simulink model "ugvGNC_complete"  (R2019a)
settings: Solver=ode45  StartTime=0.0  StopTime=200  RelTol=1e-3
InitFcn:
  | UGVparameters
StopFcn:
  | myPlot(xActEst,yActEst,X_array,Y_array,rp1,rp2)
values from neighbouring files (symbols this model uses):
  b = 0.5842    [GNCparameters.m]
  bDR = b    (= 0.5842)    [GNCparameters.m]
  eTick = 900    [GNCparameters.m]
  KP1 = 10    [GNCparameters.m]
  KP2 = 10    [GNCparameters.m]
  rL = 0.052959    [GNCparameters.m]
  rp1 = 0.3    [GNCparameters.m]
  rp2 = 0.5    [GNCparameters.m]
  rR = 0.052959    [GNCparameters.m]
  Tau1 = 0.01    [GNCparameters.m]
  Tau2 = 0.1    [GNCparameters.m]
  TauEncoderDR = 0.1    [GNCparameters.m]
  Tsample = 1/10    (= 0.1)    [GNCparameters.m]
  TsampleEncoder = 0.1    [GNCparameters.m]
  TsampleEncoderDR = TsampleEncoder    (= 0.1)    [GNCparameters.m]
  Vcom = 3*Vmax/4    (= 0.33)    [GNCparameters.m]
  wmax = Vmax/rR    (= 8.30831397874)    [GNCparameters.m]
  X_array = [3 6 6 3 0 0]    [GNCparameters.m]
  Y_array = [5 0 13 8 13 0]    [GNCparameters.m]
undefined symbols (not defined in the file or in its folder): DiscIntNeverNeededParam
libraries: simulink x12
settings Model: Creator=vigal  LastModifiedBy=lalit
settings DataIOCC: ReturnWorkspaceOutputs=off
settings DebuggingCC: ArithmeticOperatorsInVariantConditions=warning
settings SFSimCC: SimUseLocalCustomCode=off
settings RTWCC: RTWUseLocalCustomCode=off

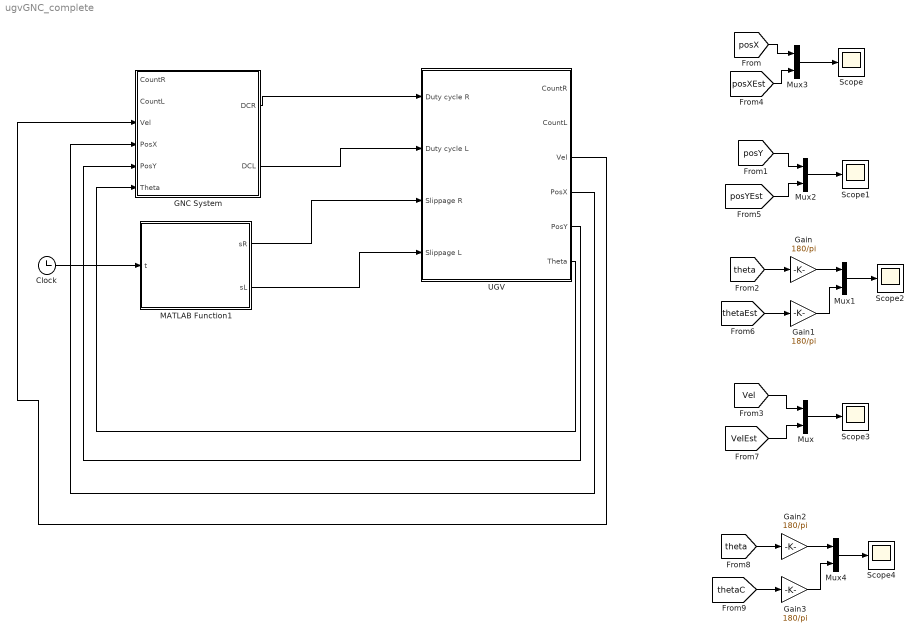
== system ugvGNC_complete ==
  Clock : Clock
  GNC System : Subsystem
  Gain{,1..3} (4 alike) : Gain  Gain=180/pi
  MATLAB Function1 : MATLAB Function  TreatAsAtomicUnit=on
  Mux{,1..4} (5 alike) : Mux  Inputs=2
  Scope{,1..4} (5 alike) : Scope
  UGV : Subsystem
  wires:
  Clock/1 -> MATLAB Function1/1(t)
  MATLAB Function1/1(sR) -> UGV/3(Slippage R)
  MATLAB Function1/2(sL) -> UGV/4(Slippage L)
  [theta] -> Gain/1
  [posX] -> Mux3/1
  [posXEst] -> Mux3/2
  Mux3/1 -> Scope/1
  Mux2/1 -> Scope1/1
  [posY] -> Mux2/1
  [posYEst] -> Mux2/2
  Gain/1 -> Mux1/1
  Mux1/1 -> Scope2/1
  [thetaEst] -> Gain1/1
  [Vel] -> Mux/1
  [VelEst] -> Mux/2
  Mux/1 -> Scope3/1
  Gain1/1 -> Mux1/2
  GNC System/1(DCR) -> UGV/1(Duty cycle R)
  GNC System/2(DCL) -> UGV/2(Duty cycle L)
  Gain3/1 -> Mux4/2
  [thetaC] -> Gain3/1
  Mux4/1 -> Scope4/1
  [theta] -> Gain2/1
  Gain2/1 -> Mux4/1
  UGV/3(Vel) -> GNC System/3(Vel)
  UGV/4(PosX) -> GNC System/4(PosX)
  UGV/5(PosY) -> GNC System/5(PosY)
  UGV/6(Theta) -> GNC System/6(Theta)

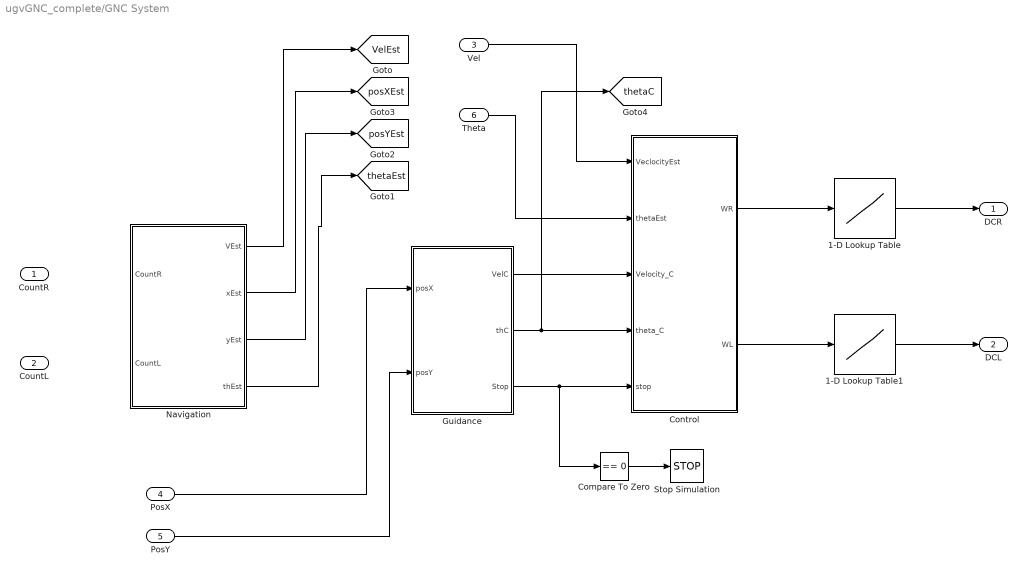
== system ugvGNC_complete/GNC System ==
  CountR : Inport
  CountL : Inport  Port=2
  Vel : Inport  Port=3
  PosX : Inport  Port=4
  PosY : Inport  Port=5
  Theta : Inport  Port=6
  1-D Lookup Table : Lookup_n-D  NumberOfTableDimensions=1  BreakpointsForDimension1=[-wmax -wmax/100 0 wmax/100 wmax]  Table=[-100 -30 0 30 100]  InternalRulePriority=Speed  RndMeth=Simplest  InputSameDT=on
  1-D Lookup Table1 : Lookup_n-D  NumberOfTableDimensions=1  BreakpointsForDimension1=[-wmax -wmax/100 0 wmax/100 wmax]  Table=[-100 -30 0 30 100]  InternalRulePriority=Speed  RndMeth=Simplest  InputSameDT=on
  Compare To Zero : simulink/Logic and Bit Operations/Compare To Zero  relop===  OutDataTypeStr=boolean
  Control : Subsystem
  Guidance : Subsystem
  Navigation : Subsystem
  Stop Simulation : Stop
  DCR : Outport
  DCL : Outport  Port=2
  tag scope: VelEst=global, posXEst=global, posYEst=global, thetaC=global, thetaEst=global
  wires:
  Navigation/1(VEst) -> [VelEst]
  Navigation/2(xEst) -> [posXEst]
  Navigation/3(yEst) -> [posYEst]
  Navigation/4(thEst) -> [thetaEst]
  Guidance/1(VelC) -> Control/3(Velocity_C)
  Guidance/2(thC) -> [thetaC], Control/4(theta_C)
  Guidance/3(Stop) -> Compare To Zero/1, Control/5(stop)
  Control/1(WR) -> 1-D Lookup Table/1
  Control/2(WL) -> 1-D Lookup Table1/1
  Compare To Zero/1 -> Stop Simulation/1
  PosX/1 -> Guidance/1(posX)
  PosY/1 -> Guidance/2(posY)
  Theta/1 -> Control/2(thetaEst)
  Vel/1 -> Control/1(VeclocityEst)
  1-D Lookup Table/1 -> DCR/1
  1-D Lookup Table1/1 -> DCL/1

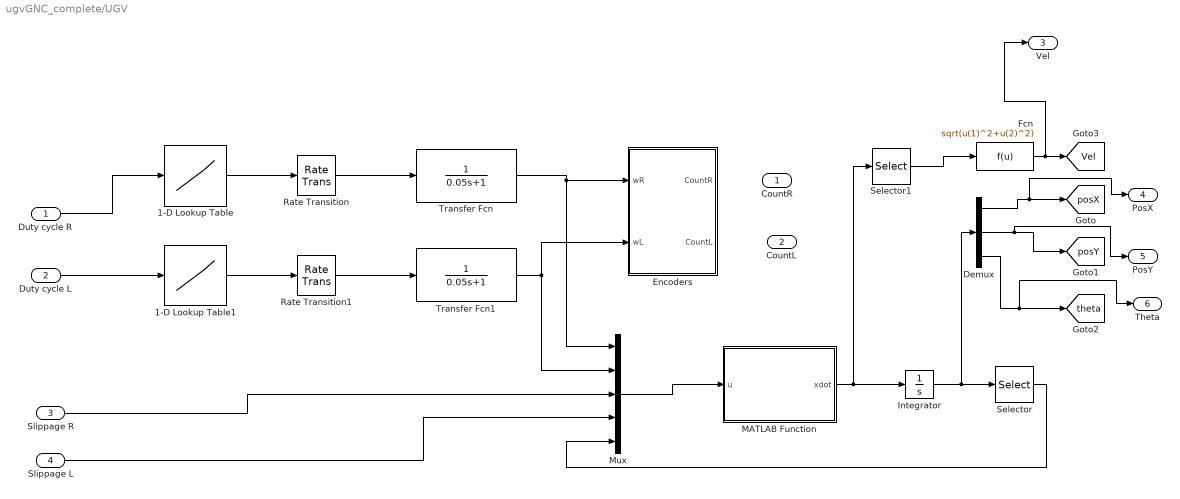
== system ugvGNC_complete/UGV ==
  Duty cycle R : Inport
  Duty cycle L : Inport  Port=2
  Slippage R : Inport  Port=3
  Slippage L : Inport  Port=4
  1-D Lookup Table : Lookup_n-D  NumberOfTableDimensions=1  BreakpointsForDimension1=[-100 -30 0 30 100]  Table=[-wmax 0 0 0 wmax]  InternalRulePriority=Speed  RndMeth=Simplest  InputSameDT=on
  1-D Lookup Table1 : Lookup_n-D  NumberOfTableDimensions=1  BreakpointsForDimension1=[-100 -30 0 30 100]  Table=[-wmax 0 0 0 wmax]  InternalRulePriority=Speed  RndMeth=Simplest  InputSameDT=on
  Demux : Demux  Outputs=3
  Encoders : Subsystem
  Fcn : Fcn  Expr=sqrt(u(1)^2+u(2)^2)
  Integrator : Integrator  InitialCondition=[0;0;0]
  MATLAB Function : MATLAB Function  TreatAsAtomicUnit=on
  Mux : Mux  Inputs=5
  Rate Transition : RateTransition
  Rate Transition1 : RateTransition
  Selector : Selector  InputPortWidth=3  IndexOptions=Index vector (dialog)  Indices=[3]  OutputSizes=1
  Selector1 : Selector  InputPortWidth=3  IndexOptions=Index vector (dialog)  Indices=[1 2]  OutputSizes=1
  Transfer Fcn : TransferFcn  Denominator=[0.05 1]
  Transfer Fcn1 : TransferFcn  Denominator=[0.05 1]
  CountR : Outport
  CountL : Outport  Port=2
  Vel : Outport  Port=3
  PosX : Outport  Port=4
  PosY : Outport  Port=5
  Theta : Outport  Port=6
  tag scope: Vel=global, posX=global, posY=global, theta=global
  wires:
  Slippage R/1 -> Mux/3
  1-D Lookup Table/1 -> Rate Transition/1
  Duty cycle R/1 -> 1-D Lookup Table/1
  Duty cycle L/1 -> 1-D Lookup Table1/1
  1-D Lookup Table1/1 -> Rate Transition1/1
  Rate Transition1/1 -> Transfer Fcn1/1
  Rate Transition/1 -> Transfer Fcn/1
  Transfer Fcn/1 -> Encoders/1(wR), Mux/1
  Slippage L/1 -> Mux/4
  Transfer Fcn1/1 -> Encoders/2(wL), Mux/2
  Mux/1 -> MATLAB Function/1(u)
  Integrator/1 -> Demux/1, Selector/1
  Selector/1 -> Mux/5
  Demux/1 -> PosX/1, [posX]
  Demux/3 -> Theta/1, [theta]
  Demux/2 -> PosY/1, [posY]
  MATLAB Function/1(xdot) -> Selector1/1, Integrator/1
  Selector1/1 -> Fcn/1
  Fcn/1 -> Vel/1, [Vel]

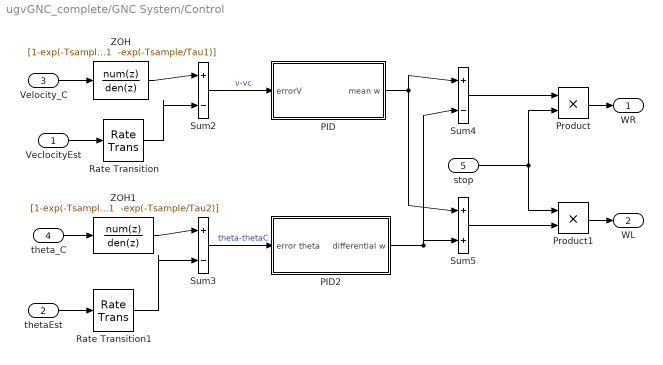
== system ugvGNC_complete/GNC System/Control ==
  VeclocityEst : Inport
  thetaEst : Inport  Port=2
  Velocity_C : Inport  Port=3
  theta_C : Inport  Port=4
  stop : Inport  Port=5
  PID : Subsystem
  PID2 : Subsystem
  Product : Product  RndMeth=Zero
  Product1 : Product  RndMeth=Zero
  Rate Transition : RateTransition  Deterministic=off
  Rate Transition1 : RateTransition  Deterministic=off
  Sum2 : Sum  Inputs=|+|-|  SampleTime=Tsample
  Sum3 : Sum  Inputs=|+|-|  SampleTime=Tsample
  Sum4 : Sum  Inputs=+|-
  Sum5 : Sum  Inputs=+|+
  ZOH : DiscreteTransferFcn  Numerator=[1-exp(-Tsample/Tau1)]  Denominator="[1  -exp(-Tsample/Tau1)]"  SampleTime=Tsample
  ZOH1 : DiscreteTransferFcn  Numerator=[1-exp(-Tsample/Tau2)]  Denominator="[1  -exp(-Tsample/Tau2)]"  SampleTime=Tsample
  WR : Outport
  WL : Outport  Port=2
  wires:
  Product1/1 -> WL/1
  Product/1 -> WR/1
  Sum5/1 -> Product1/2
  stop/1 -> Product/2, Product1/1
  Sum4/1 -> Product/1
  PID2/1(differential w) -> Sum5/2, Sum4/2
  PID/1(mean w) -> Sum5/1, Sum4/1
  theta_C/1 -> ZOH1/1
  thetaEst/1 -> Rate Transition1/1
  Velocity_C/1 -> ZOH/1
  VeclocityEst/1 -> Rate Transition/1
  Sum2/1 -> PID/1(errorV)  "v-vc"
  Sum3/1 -> PID2/1(error theta)  "theta-thetaC"
  ZOH/1 -> Sum2/1
  Rate Transition/1 -> Sum2/2
  ZOH1/1 -> Sum3/1
  Rate Transition1/1 -> Sum3/2

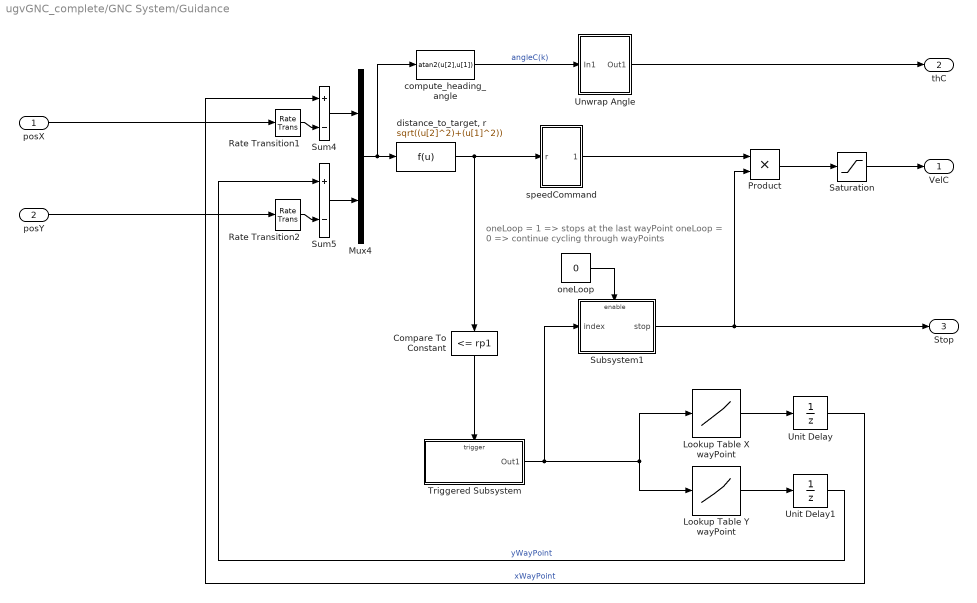
== system ugvGNC_complete/GNC System/Guidance ==
  note: oneLoop = 1 => stops at the last wayPoint
      | oneLoop = 0 => continue cycling through wayPoints
  posX : Inport
  posY : Inport  Port=2
  Compare To Constant : simulink/Logic and Bit Operations/Compare To Constant  relop=<=  const=rp1  OutDataTypeStr=uint8  ZeroCross=off
  Lookup Table X wayPoint : Lookup  InputValues=[1:length(X_array)]  Table=X_array  LookUpMeth=Interpolation-Use End Values  OutDataTypeStr=double
  Lookup Table Y wayPoint : Lookup  InputValues=[1:length(Y_array)]  Table=Y_array  LookUpMeth=Interpolation-Use End Values  OutDataTypeStr=double
  Mux4 : Mux  Inputs=2
  Product : Product  RndMeth=Zero
  Rate Transition1 : RateTransition
  Rate Transition2 : RateTransition
  Saturation : Saturate  UpperLimit=Vcom  LowerLimit=0  SampleTime=Tsample
  Subsystem1 : Subsystem
  Sum4 : Sum  Inputs=|+|-|
  Sum5 : Sum  Inputs=|+|-|
  Triggered Subsystem : Subsystem  TreatAsAtomicUnit=on
  Unit Delay : UnitDelay  SampleTime=Tsample  HasFrameUpgradeWarning=on
  Unit Delay1 : UnitDelay  SampleTime=Tsample  HasFrameUpgradeWarning=on
  Unwrap Angle : Subsystem
  compute_heading_angle : Fcn  Expr=atan2(u[2],u[1])  SampleTime=Tsample
  "distance_to_target, r" : Fcn  Expr=sqrt((u[2]^2)+(u[1]^2))  SampleTime=Tsample
  oneLoop : Constant  Value=0  OutDataTypeStr=uint32  SampleTime=Tsample
  speedCommand : Subsystem
  VelC : Outport
  thC : Outport  Port=2
  Stop : Outport  Port=3
  wires:
  Compare To Constant/1 -> Triggered Subsystem/Trigger
  oneLoop/1 -> Subsystem1/Enable
  Sum5/1 -> Mux4/2
  Unit Delay/1 -> Sum4/1  "xWayPoint"
  Triggered Subsystem/1(Out1) -> Subsystem1/1(index), Lookup Table X wayPoint/1, Lookup Table Y wayPoint/1
  Lookup Table Y wayPoint/1 -> Unit Delay1/1
  Sum4/1 -> Mux4/1
  Subsystem1/1(stop) -> Stop/1, Product/2
  Product/1 -> Saturation/1
  Rate Transition1/1 -> Sum4/2
  Unit Delay1/1 -> Sum5/1  "yWayPoint"
  posX/1 -> Rate Transition1/1
  posY/1 -> Rate Transition2/1
  Mux4/1 -> "distance_to_target, r"/1, compute_heading_angle/1
  Lookup Table X wayPoint/1 -> Unit Delay/1
  Rate Transition2/1 -> Sum5/2
  compute_heading_angle/1 -> Unwrap Angle/1(In1)  "angleC(k)"
  "distance_to_target, r"/1 -> Compare To Constant/1, speedCommand/1(r)
  speedCommand/1(Vdes) -> Product/1
  Saturation/1 -> VelC/1
  Unwrap Angle/1(Out1) -> thC/1

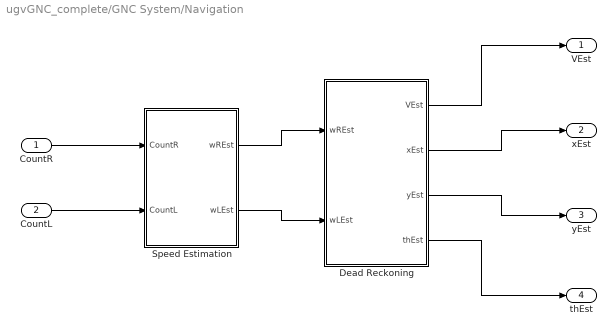
== system ugvGNC_complete/GNC System/Navigation ==
  CountR : Inport
  CountL : Inport  Port=2
  Dead Reckoning : Subsystem
  Speed Estimation : Subsystem
  VEst : Outport
  xEst : Outport  Port=2
  yEst : Outport  Port=3
  thEst : Outport  Port=4
  wires:
  Dead Reckoning/1(VEst) -> VEst/1
  Dead Reckoning/3(yEst) -> yEst/1
  Speed Estimation/2(wLEst) -> Dead Reckoning/2(wLEst)
  CountR/1 -> Speed Estimation/1(CountR)
  Dead Reckoning/2(xEst) -> xEst/1
  CountL/1 -> Speed Estimation/2(CountL)
  Speed Estimation/1(wREst) -> Dead Reckoning/1(wREst)
  Dead Reckoning/4(thEst) -> thEst/1

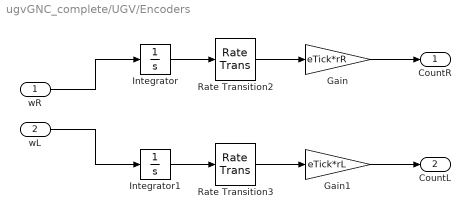
== system ugvGNC_complete/UGV/Encoders ==
  wR : Inport
  wL : Inport  Port=2
  Gain : Gain  Gain=eTick*rR  OutDataTypeStr=int16
  Gain1 : Gain  Gain=eTick*rL  OutDataTypeStr=int16
  Integrator : Integrator
  Integrator1 : Integrator
  Rate Transition2 : RateTransition  OutPortSampleTime=TsampleEncoder
  Rate Transition3 : RateTransition  OutPortSampleTime=TsampleEncoder
  CountR : Outport
  CountL : Outport  Port=2
  wires:
  Integrator1/1 -> Rate Transition3/1
  Integrator/1 -> Rate Transition2/1
  Gain1/1 -> CountL/1
  Rate Transition3/1 -> Gain1/1
  Rate Transition2/1 -> Gain/1
  Gain/1 -> CountR/1
  wR/1 -> Integrator/1
  wL/1 -> Integrator1/1

== system ugvGNC_complete/GNC System/Control/PID ==
  errorV : Inport
  Discrete Derivative : simulink/Discrete/Discrete Derivative  gainval=KD1  ICPrevScaledInput=0.0  OutMin=[]  OutMax=[]  OutDataType=sfix(16)  OutScaling=2^-10  DoSatur=off
  Discrete-Time Integrator : DiscreteIntegrator  gainval=KI1  SampleTime=Tsample  ICPrevOutput=DiscIntNeverNeededParam  ICPrevScaledInput=DiscIntNeverNeededParam
  Gain : Gain  Gain=KP1  SampleTime=Tsample
  Sum : Sum  Inputs=+|+|+
  Zero-Order Hold : ZeroOrderHold  SampleTime=Tsample
  mean w : Outport
  wires:
  Discrete Derivative/1 -> Sum/3
  Zero-Order Hold/1 -> Discrete Derivative/1
  Discrete-Time Integrator/1 -> Sum/2
  Gain/1 -> Sum/1
  errorV/1 -> Discrete-Time Integrator/1, Gain/1, Zero-Order Hold/1
  Sum/1 -> mean w/1

== system ugvGNC_complete/GNC System/Control/PID2 ==
  error theta : Inport
  Discrete Derivative1 : simulink/Discrete/Discrete Derivative  gainval=KD2  ICPrevScaledInput=0.0  OutMin=[]  OutMax=[]  OutDataType=sfix(16)  OutScaling=2^-10  DoSatur=off
  Discrete-Time Integrator1 : DiscreteIntegrator  gainval=KI2  SampleTime=Tsample  ICPrevOutput=DiscIntNeverNeededParam  ICPrevScaledInput=DiscIntNeverNeededParam
  Gain1 : Gain  Gain=KP2  SampleTime=Tsample
  Sum1 : Sum  Inputs=+|+|+
  Zero-Order Hold1 : ZeroOrderHold  SampleTime=Tsample
  differential w : Outport
  wires:
  Discrete Derivative1/1 -> Sum1/3
  Zero-Order Hold1/1 -> Discrete Derivative1/1
  error theta/1 -> Gain1/1, Discrete-Time Integrator1/1, Zero-Order Hold1/1
  Discrete-Time Integrator1/1 -> Sum1/2
  Gain1/1 -> Sum1/1
  Sum1/1 -> differential w/1

== system ugvGNC_complete/GNC System/Guidance/Subsystem1 ==
  note: NAND = TRUE
      | if at least one input is FALSE
  index : Inport
  Enable : EnablePort
  Compare To Constant1 : simulink/Logic and Bit Operations/Compare To Constant  relop===  const=1  OutDataTypeStr=uint8  ZeroCross=off
  Compare To Constant2 : simulink/Logic and Bit Operations/Compare To Constant  relop===  const=length(X_array)  OutDataTypeStr=uint8  ZeroCross=off
  Logical Operator1 : Logic  Operator=NAND  IconShape=distinctive  AllPortsSameDT=off  OutDataTypeStr=boolean
  Triggered Subsystem2 : Subsystem  TreatAsAtomicUnit=on
  stop : Outport  OutputWhenDisabled=reset  InitialOutput=[1]
  wires:
  Logical Operator1/1 -> stop/1
  index/1 -> Compare To Constant1/1, Compare To Constant2/1
  Compare To Constant1/1 -> Logical Operator1/1
  Triggered Subsystem2/1(Out1) -> Logical Operator1/2
  Compare To Constant2/1 -> Triggered Subsystem2/Trigger

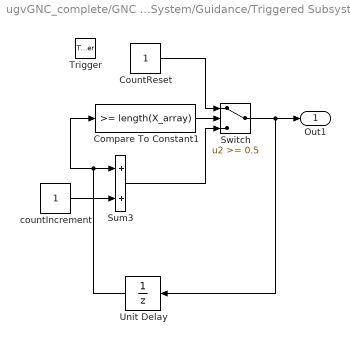
== system ugvGNC_complete/GNC System/Guidance/Triggered Subsystem ==
  Trigger : TriggerPort  VariantControl=(inherit)
  Compare To Constant1 : simulink/Logic and Bit Operations/Compare To Constant  relop=>=  const=length(X_array)  OutDataTypeStr=uint8  ZeroCross=off
  CountReset : Constant  OutDataTypeStr=uint32  SampleTime=-1
  Sum3 : Sum  OutDataTypeStr=uint32
  Switch : Switch  Threshold=0.5
  Unit Delay : UnitDelay  InitialCondition=1  SampleTime=-1  HasFrameUpgradeWarning=on
  countIncrement : Constant  OutDataTypeStr=uint32  SampleTime=-1
  Out1 : Outport  OutDataTypeStr=uint32  InitialOutput=1
  wires:
  countIncrement/1 -> Sum3/2
  Unit Delay/1 -> Compare To Constant1/1, Sum3/1
  Compare To Constant1/1 -> Switch/2
  Switch/1 -> Out1/1, Unit Delay/1
  CountReset/1 -> Switch/1
  Sum3/1 -> Switch/3

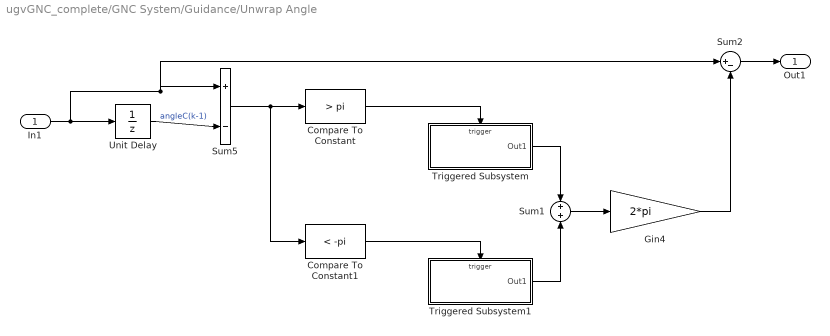
== system ugvGNC_complete/GNC System/Guidance/Unwrap Angle ==
  In1 : Inport
  Compare To Constant : simulink/Logic and Bit Operations/Compare To Constant  relop=>  const=pi  OutDataTypeStr=uint8  ZeroCross=off
  Compare To Constant1 : simulink/Logic and Bit Operations/Compare To Constant  relop=<  const=-pi  OutDataTypeStr=uint8  ZeroCross=off
  Gin4 : Gain  Gain=2*pi  OutDataTypeStr=double  SampleTime=Tsample
  Sum1 : Sum  Inputs=+|+
  Sum2 : Sum  Inputs=|+-
  Sum5 : Sum  Inputs=|+|-|
  Triggered Subsystem : Subsystem  TreatAsAtomicUnit=on
  Triggered Subsystem1 : Subsystem  TreatAsAtomicUnit=on
  Unit Delay : UnitDelay  SampleTime=Tsample  HasFrameUpgradeWarning=on
  Out1 : Outport
  wires:
  In1/1 -> Unit Delay/1, Sum5/1, Sum2/1
  Unit Delay/1 -> Sum5/2  "angleC(k-1)"
  Sum5/1 -> Compare To Constant/1, Compare To Constant1/1
  Compare To Constant1/1 -> Triggered Subsystem1/Trigger
  Compare To Constant/1 -> Triggered Subsystem/Trigger
  Triggered Subsystem/1(Out1) -> Sum1/1
  Triggered Subsystem1/1(Out1) -> Sum1/2
  Sum1/1 -> Gin4/1
  Sum2/1 -> Out1/1
  Gin4/1 -> Sum2/2

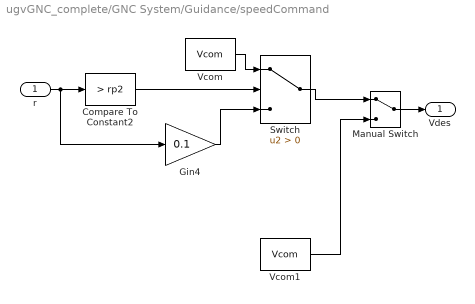
== system ugvGNC_complete/GNC System/Guidance/speedCommand ==
  r : Inport
  Compare To Constant2 : simulink/Logic and Bit Operations/Compare To Constant  relop=>  const=rp2  OutDataTypeStr=uint8  ZeroCross=off
  Gin4 : Gain  Gain=0.1  SampleTime=Tsample
  Manual Switch : ManualSwitch
  Switch : Switch  Criteria=u2 > Threshold
  Vcom : Constant  Value=Vcom  SampleTime=Tsample
  Vcom1 : Constant  Value=Vcom  SampleTime=Tsample
  Vdes : Outport
  wires:
  Compare To Constant2/1 -> Switch/2
  Vcom/1 -> Switch/1
  Vcom1/1 -> Manual Switch/2
  Switch/1 -> Manual Switch/1
  Gin4/1 -> Switch/3
  r/1 -> Compare To Constant2/1, Gin4/1
  Manual Switch/1 -> Vdes/1

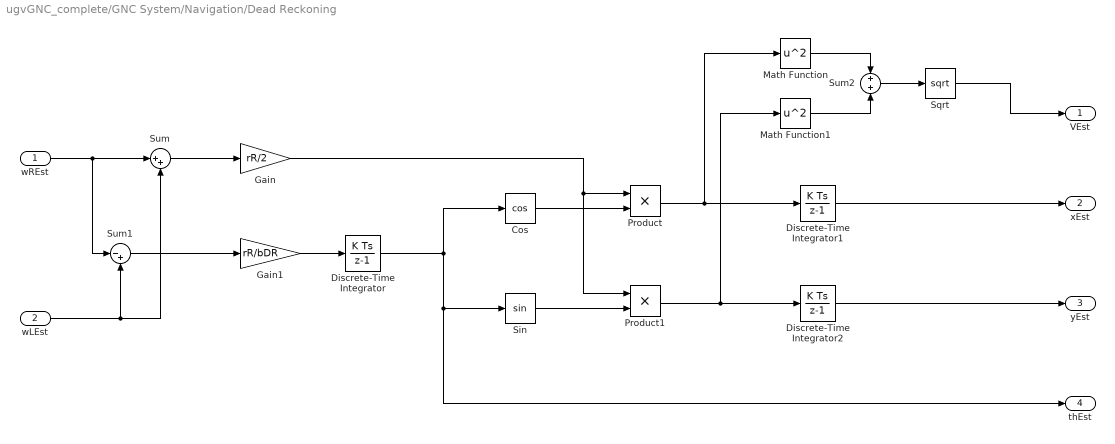
== system ugvGNC_complete/GNC System/Navigation/Dead Reckoning ==
  wREst : Inport
  wLEst : Inport  Port=2
  Cos : Trigonometry  Operator=cos
  Discrete-Time Integrator : DiscreteIntegrator  SampleTime=-1  OutDataTypeStr=double  ICPrevOutput=DiscIntNeverNeededParam  ICPrevScaledInput=DiscIntNeverNeededParam
  Discrete-Time Integrator1 : DiscreteIntegrator  SampleTime=-1  OutDataTypeStr=double  ICPrevOutput=DiscIntNeverNeededParam  ICPrevScaledInput=DiscIntNeverNeededParam
  Discrete-Time Integrator2 : DiscreteIntegrator  SampleTime=-1  OutDataTypeStr=double  ICPrevOutput=DiscIntNeverNeededParam  ICPrevScaledInput=DiscIntNeverNeededParam
  Gain : Gain  Gain=rR/2
  Gain1 : Gain  Gain=rR/bDR
  Math Function : Math  Operator=square  SaturateOnIntegerOverflow=on
  Math Function1 : Math  Operator=square  SaturateOnIntegerOverflow=on
  Product : Product
  Product1 : Product
  Sin : Trigonometry
  Sqrt : Sqrt  SaturateOnIntegerOverflow=on
  Sum : Sum  Inputs=|++
  Sum1 : Sum  Inputs=|-+
  Sum2 : Sum  Inputs=+|+
  VEst : Outport
  xEst : Outport  Port=2
  yEst : Outport  Port=3
  thEst : Outport  Port=4
  wires:
  wLEst/1 -> Sum1/2, Sum/2
  wREst/1 -> Sum1/1, Sum/1
  Sum/1 -> Gain/1
  Sum1/1 -> Gain1/1
  Gain1/1 -> Discrete-Time Integrator/1
  Discrete-Time Integrator/1 -> thEst/1, Sin/1, Cos/1
  Cos/1 -> Product/2
  Sin/1 -> Product1/2
  Gain/1 -> Product1/1, Product/1
  Product/1 -> Math Function/1, Discrete-Time Integrator1/1
  Product1/1 -> Math Function1/1, Discrete-Time Integrator2/1
  Math Function/1 -> Sum2/1
  Math Function1/1 -> Sum2/2
  Sum2/1 -> Sqrt/1
  Sqrt/1 -> VEst/1
  Discrete-Time Integrator1/1 -> xEst/1
  Discrete-Time Integrator2/1 -> yEst/1

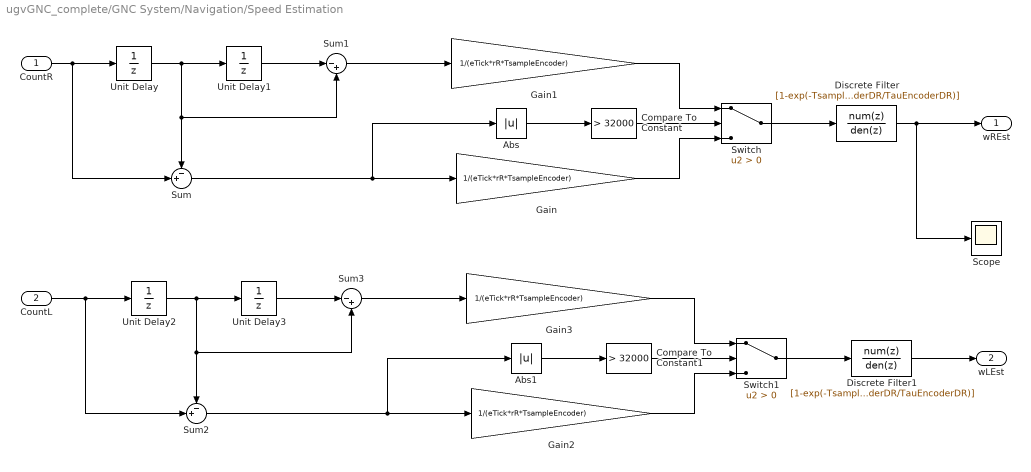
== system ugvGNC_complete/GNC System/Navigation/Speed Estimation ==
  CountR : Inport
  CountL : Inport  Port=2
  Abs : Abs
  Abs1 : Abs
  Compare To Constant : simulink/Logic and Bit Operations/Compare To Constant  relop=>  const=32000  OutDataTypeStr=boolean
  Compare To Constant1 : simulink/Logic and Bit Operations/Compare To Constant  relop=>  const=32000  OutDataTypeStr=boolean
  Discrete Filter : DiscreteFilter  Numerator=[1-exp(-TsampleEncoderDR/TauEncoderDR)]  Denominator=[1 -exp(-TsampleEncoderDR/TauEncoderDR)]
  Discrete Filter1 : DiscreteFilter  Numerator=[1-exp(-TsampleEncoderDR/TauEncoderDR)]  Denominator=[1 -exp(-TsampleEncoderDR/TauEncoderDR)]
  Gain{,1..3} (4 alike) : Gain  Gain=1/(eTick*rR*TsampleEncoder)
  Scope : Scope
  Sum : Sum  Inputs=-+|
  Sum1 : Sum  Inputs=|-+
  Sum2 : Sum  Inputs=-+|
  Sum3 : Sum  Inputs=|-+
  Switch : Switch  Criteria=u2 > Threshold
  Switch1 : Switch  Criteria=u2 > Threshold
  Unit Delay{,1..3} (4 alike) : UnitDelay  SampleTime=-1  HasFrameUpgradeWarning=on
  wREst : Outport
  wLEst : Outport  Port=2
  wires:
  Unit Delay/1 -> Sum1/2, Sum/1, Unit Delay1/1
  CountR/1 -> Sum/2, Unit Delay/1
  Unit Delay1/1 -> Sum1/1
  Sum/1 -> Abs/1, Gain/1
  Sum1/1 -> Gain1/1
  Abs/1 -> Compare To Constant/1
  Compare To Constant/1 -> Switch/2
  Gain/1 -> Switch/3
  Gain1/1 -> Switch/1
  Switch/1 -> Discrete Filter/1
  Discrete Filter/1 -> Scope/1, wREst/1
  Unit Delay2/1 -> Sum3/2, Sum2/1, Unit Delay3/1
  Unit Delay3/1 -> Sum3/1
  Sum3/1 -> Gain3/1
  CountL/1 -> Sum2/2, Unit Delay2/1
  Sum2/1 -> Abs1/1, Gain2/1
  Compare To Constant1/1 -> Switch1/2
  Discrete Filter1/1 -> wLEst/1
  Gain3/1 -> Switch1/1
  Switch1/1 -> Discrete Filter1/1
  Gain2/1 -> Switch1/3
  Abs1/1 -> Compare To Constant1/1

== system ugvGNC_complete/GNC System/Guidance/Subsystem1/Triggered Subsystem2 ==
  Trigger : TriggerPort  VariantControl=(inherit)
  Constant : Constant  OutDataTypeStr=uint32  SampleTime=-1
  Out1 : Outport  OutDataTypeStr=uint32  InitialOutput=0
  wires:
  Constant/1 -> Out1/1

== system ugvGNC_complete/GNC System/Guidance/Unwrap Angle/Triggered Subsystem ==
  Trigger : TriggerPort  VariantControl=(inherit)
  Sum3 : Sum  OutDataTypeStr=int32
  Unit Delay : UnitDelay  SampleTime=-1  HasFrameUpgradeWarning=on
  countIncrement : Constant  OutDataTypeStr=int32  SampleTime=-1
  Out1 : Outport  OutDataTypeStr=int32  InitialOutput=0
  wires:
  countIncrement/1 -> Sum3/2
  Unit Delay/1 -> Sum3/1
  Sum3/1 -> Out1/1, Unit Delay/1

== system ugvGNC_complete/GNC System/Guidance/Unwrap Angle/Triggered Subsystem1 ==
  Trigger : TriggerPort  VariantControl=(inherit)
  Sum3 : Sum  Inputs=+-  OutDataTypeStr=int32
  Unit Delay : UnitDelay  SampleTime=-1  HasFrameUpgradeWarning=on
  countIncrement : Constant  OutDataTypeStr=int32  SampleTime=-1
  Out1 : Outport  OutDataTypeStr=int32  InitialOutput=0
  wires:
  Sum3/1 -> Out1/1, Unit Delay/1
  Unit Delay/1 -> Sum3/1
  countIncrement/1 -> Sum3/2

== matlab function ugvGNC_complete/MATLAB Function1 ==
  data: t input; sR output; sL output
function [sR,sL] = slip(t)
%Simulation of the slippage factor on wheels

sR=0;
sL=0;

if t>50 && t<60
    sR=0.2;
    sL=0;
end

== matlab function ugvGNC_complete/UGV/MATLAB Function ==
  data: u input; xdot output; rR parameter; rL parameter; b parameter
function xdot = ugv(u,rR, rL, b)

wR=u(1);
wL=u(2);
sR=u(3);
sL=u(4);
theta=u(5);

xdot=[((1-sL)*rL*wL+(1-sR)*rR*wR)*cos(theta)/2;...
       ((1-sL)*rL*wL+(1-sR)*rR*wR)*sin(theta)/2;...
       ((1-sL)*rL*wL-(1-sR)*rR*wR)/b];
